simulink model "KF_Model_Double"  (R2024b)
settings: Solver=FixedStepDiscrete  StartTime=0.0  StopTime=0.1  FixedStep=1e-5  RelTol=1e-3
libraries: dspsrcs4 x3
settings Model: Creator=bzwan  LastModifiedBy=bzwan
settings OptimizationCC: UseDivisionForNetSlopeComputation=on
settings HardwareCC: ProdBitPerPointer=32  ProdBitPerSizeT=32  ProdBitPerPtrDiffT=32  ProdLargestAtomicFloat=None  ProdIntDivRoundTo=Undefined  ProdEndianess=Unspecified  ProdWordSize=32  ProdHWDeviceType=ASIC/FPGA->ASIC/FPGA  TargetBitPerPointer=64  TargetBitPerSizeT=64  TargetBitPerPtrDiffT=64  TargetLongLongMode=on  TargetIntDivRoundTo=Zero  TargetEndianess=LittleEndian  TargetWordSize=64  TargetHWDeviceType=Custom Processor->MATLAB Host Computer  ProdEqTarget=off

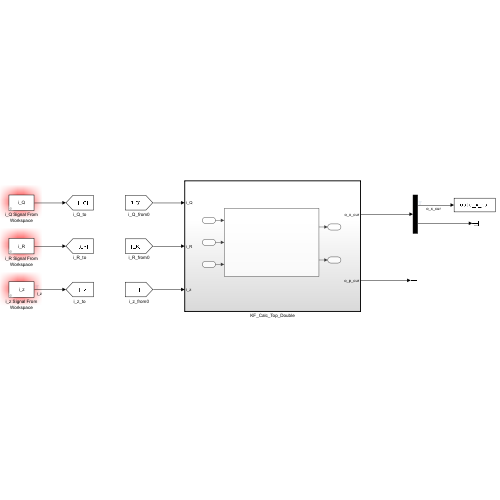
[thumbnail: Simulink's stored preview of the top-level diagram]
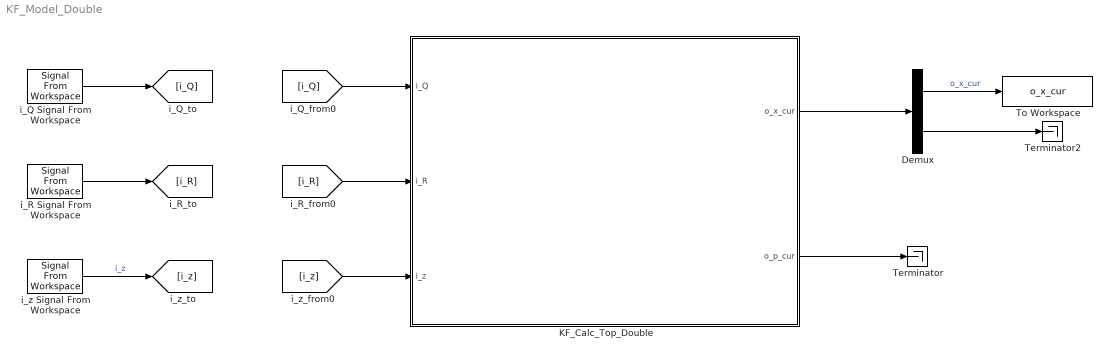
== system KF_Model_Double ==
  Demux : Demux  Outputs=2
  KF_Calc_Top_Double : Subsystem  TreatAsAtomicUnit=on  SystemSampleTime=1/10000
  Terminator : Terminator
  Terminator2 : Terminator
  To Workspace : ToWorkspace  VariableName=o_x_cur  SaveFormat=Structure  SampleTime=-1
  i_Q Signal From Workspace : dspsrcs4/Signal From Workspace  X=i_Q  Ts=1/10000  nsamps=1  OutputAfterFinalValue=Cyclic repetition  ignoreOrWarnInputAndFrameLengths=off  OutputFrames=off
  i_R Signal From Workspace : dspsrcs4/Signal From Workspace  X=i_R  Ts=1/10000  nsamps=1  OutputAfterFinalValue=Cyclic repetition  ignoreOrWarnInputAndFrameLengths=off  OutputFrames=off
  i_z Signal From Workspace : dspsrcs4/Signal From Workspace  X=i_z  Ts=1/10000  nsamps=1  OutputAfterFinalValue=Cyclic repetition  ignoreOrWarnInputAndFrameLengths=off  OutputFrames=off
  wires:
  KF_Calc_Top_Double/1(o_x_cur) -> Demux/1
  KF_Calc_Top_Double/2(o_p_cur) -> Terminator/1
  i_z Signal From Workspace/1 -> [i_z]  "i_z"
  [i_z] -> KF_Calc_Top_Double/3(i_z)
  [i_Q] -> KF_Calc_Top_Double/1(i_Q)
  i_R Signal From Workspace/1 -> [i_R]
  [i_R] -> KF_Calc_Top_Double/2(i_R)
  Demux/1 -> To Workspace/1  "o_x_cur"
  Demux/2 -> Terminator2/1
  i_Q Signal From Workspace/1 -> [i_Q]

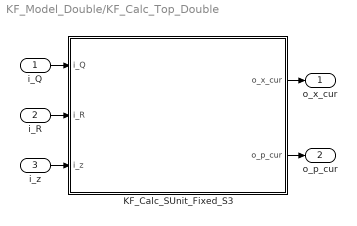
== system KF_Model_Double/KF_Calc_Top_Double ==
  i_Q : Inport
  i_R : Inport  Port=2
  i_z : Inport  Port=3
  KF_Calc_SUnit_Fixed_S3 : MATLAB Function  TreatAsAtomicUnit=on
  o_x_cur : Outport
  o_p_cur : Outport  Port=2
  wires:
  i_R/1 -> KF_Calc_SUnit_Fixed_S3/2(i_R)
  i_Q/1 -> KF_Calc_SUnit_Fixed_S3/1(i_Q)
  KF_Calc_SUnit_Fixed_S3/1(o_x_cur) -> o_x_cur/1
  i_z/1 -> KF_Calc_SUnit_Fixed_S3/3(i_z)
  KF_Calc_SUnit_Fixed_S3/2(o_p_cur) -> o_p_cur/1

== matlab function KF_Model_Double/KF_Calc_Top_Double/KF_Calc_SUnit_Fixed_S3 ==
  data: i_Q input; o_x_cur output; i_R input; i_z input; o_p_cur output
function [o_x_cur, o_p_cur]= KF_Calc_SUnit_Fixed_S3(i_Q, i_R, i_z) %#codegen
    
    % input is wire but hold as reg
    z = i_z;
    Q = i_Q;
    R = i_R;

    % reg define start
    persistent x_cur p_cur
    % reg define end
    
    if isempty(x_cur)
        x_cur = [0; 1];
    end

    if isempty(p_cur)
        p_cur = eye(2).*10;
    end

    % wire define start
    x_nxt_pre = zeros(2,1);
    x_nxt = zeros(2,1);
    p_nxt = zeros(2,2);
    k_cur_pre = zeros(2,1);
    k_cur_pos = zeros(1,1);
    k_cur_pos_inv = zeros(1,1);
    k_cur = zeros(2,1);
    x_cur_pos = zeros(1,1);
    p_cur_pre = zeros(2,2);
    % wire define end
    
    % predict
    x_nxt_pre(1,1) = (x_cur(1,1) + x_cur(2,1));
    x_nxt_pre(2,1) = x_cur(2,1);

    x_nxt(1,1) = x_nxt_pre(1,1);
    x_nxt(2,1) = x_nxt_pre(2,1);

    p_nxt(1,1) = (p_cur(1,1) + p_cur(2,1)) + ...
                 (p_cur(1,2) + p_cur(2,2)) + Q;
    p_nxt(1,2) = (p_cur(1,2) + p_cur(2,2));
    p_nxt(2,1) = (p_cur(2,1) + p_cur(2,2));
    p_nxt(2,2) = (p_cur(2,2) + Q);

    % update
    k_cur_pre(1,1) = p_nxt(1,1);
    k_cur_pre(2,1) = p_nxt(2,1);

    k_cur_pos(1,1) = (p_nxt(1,1) + R);

    if k_cur_pos(1,1) < .2e-1
        k_cur_pos(1,1) = .2e-1;
    end

    %%%%%%%%%%%%%%%%%%%%%%%%%%%%%%%%%%%%%%%%%%%%%%%%%%%%%%%
    k_cur_pos_inv(1,1) = 1/k_cur_pos(1,1);
    %%%%%%%%%%%%%%%%%%%%%%%%%%%%%%%%%%%%%%%%%%%%%%%%%%%%%%%

    k_cur(1,1) = (k_cur_pre(1,1)*k_cur_pos_inv(1,1));
    k_cur(2,1) = (k_cur_pre(2,1)*k_cur_pos_inv(1,1));

    x_cur_pos(1,1) = (z(1,1) - x_nxt(1,1));

    x_cur(1,1) = (x_nxt(1,1) + (k_cur(1,1)*x_cur_pos(1,1)));
    x_cur(2,1) = (x_nxt(2,1) + (k_cur(2,1)*x_cur_pos(1,1)));

    p_cur_pre(1,1) = (1 - k_cur(1,1));
    p_cur_pre(1,2) = 0;
    p_cur_pre(2,1) = (0 - k_cur(2,1));
    p_cur_pre(2,2) = 1;

    p_cur(1,1) = (p_cur_pre(1,1)*p_nxt(1,1) + p_cur_pre(1,2)*p_nxt(2,1));
    p_cur(1,2) = (p_cur_pre(1,1)*p_nxt(1,2) + p_cur_pre(1,2)*p_nxt(2,2));
    p_cur(2,1) = (p_cur_pre(2,1)*p_nxt(1,1) + p_cur_pre(2,2)*p_nxt(2,1));
    p_cur(2,2) = (p_cur_pre(2,1)*p_nxt(1,2) + p_cur_pre(2,2)*p_nxt(2,2));

    o_x_cur = x_cur;
    o_p_cur = p_cur;
end
